simulink model "GlobalVariableTest"  (R2020a)
settings: Solver=VariableStepAuto  StartTime=0.0  StopTime=1  RelTol=1e-3
undefined symbols (not defined in the file or in its folder): DiscIntNeverNeededParam
settings Model: Creator=robot  LastModifiedBy=robot

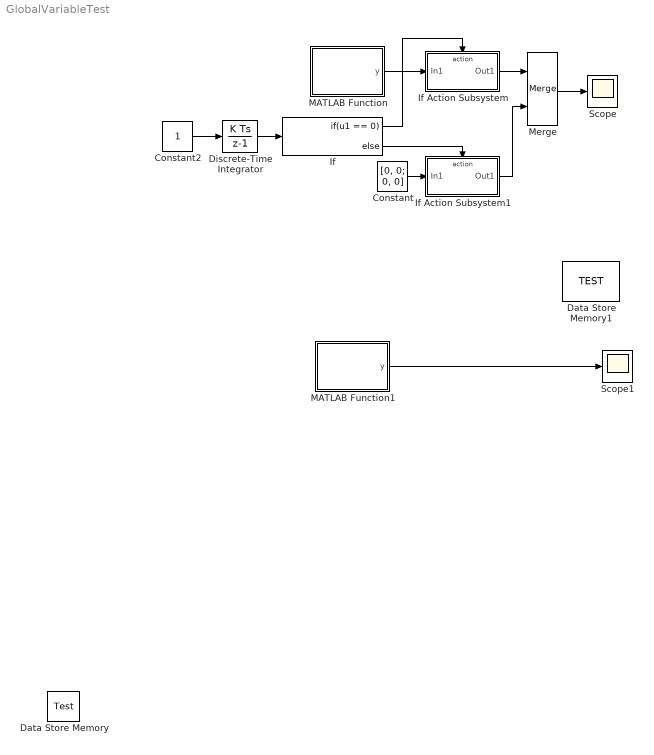
== system GlobalVariableTest ==
  Constant : Constant  Value=[0, 0; 0, 0]
  Constant2 : Constant
  Data Store Memory1 : DataStoreMemory  DataStoreName=TEST  ReadBeforeWriteMsg=warning  WriteAfterWriteMsg=warning  WriteAfterReadMsg=warning  VectorParams1D=off  ShowAdditionalParam=off  OutDataTypeStr=double  Dimensions=[2 ;2]
  Data Store Memory : DataStoreMemory  DataStoreName=Test  ReadBeforeWriteMsg=warning  WriteAfterWriteMsg=warning  WriteAfterReadMsg=warning  ShowAdditionalParam=off
  Discrete-Time Integrator : DiscreteIntegrator  SampleTime=-1  ICPrevOutput=DiscIntNeverNeededParam  ICPrevScaledInput=DiscIntNeverNeededParam
  If : If  IfExpression=u1 == 0
  If Action Subsystem : Subsystem  TreatAsAtomicUnit=on
  If Action Subsystem1 : Subsystem  TreatAsAtomicUnit=on
  MATLAB Function : MATLAB Function  TreatAsAtomicUnit=on
  MATLAB Function1 : MATLAB Function  TreatAsAtomicUnit=on
  Merge : Merge
  Scope : Scope
  Scope1 : Scope
  wires:
  MATLAB Function1/1(y) -> Scope1/1
  If/1 -> If Action Subsystem/Action
  Discrete-Time Integrator/1 -> If/1
  Constant2/1 -> Discrete-Time Integrator/1
  MATLAB Function/1(y) -> If Action Subsystem/1(In1)
  If/2 -> If Action Subsystem1/Action
  Constant/1 -> If Action Subsystem1/1(In1)
  If Action Subsystem1/1(Out1) -> Merge/2
  If Action Subsystem/1(Out1) -> Merge/1
  Merge/1 -> Scope/1

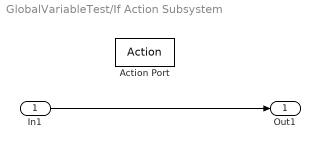
== system GlobalVariableTest/If Action Subsystem ==
  In1 : Inport
  Action Port : ActionPort  ActionPortLabel=if(u1 == 0)
  Out1 : Outport
  wires:
  In1/1 -> Out1/1

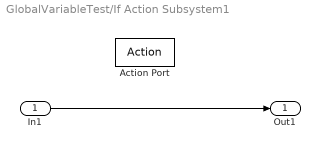
== system GlobalVariableTest/If Action Subsystem1 ==
  In1 : Inport
  Action Port : ActionPort  ActionPortLabel=else
  Out1 : Outport
  wires:
  In1/1 -> Out1/1

== matlab function GlobalVariableTest/MATLAB Function1 ==
  data: y output; TEST data_store_memory
function y = fcn
global TEST;

% y = sum(TEST, 'all');

y=TEST;

== matlab function GlobalVariableTest/MATLAB Function ==
  data: y output; TEST data_store_memory
function y = fcn
global TEST;

data = load('TestValue.mat');
TEST = data.TestValue;

y = TEST;

% y=TEST;
